simulink model "practice_main_pulse_inSimulink"  (R2019b)
settings: Solver=VariableStepAuto  StartTime=0.0  StopTime=0.1  RelTol=1e-3
InitFcn:
  | v_in=12;
undefined symbols (not defined in the file): plecs
settings Model: Creator=Nahid  LastModifiedBy=Nahid

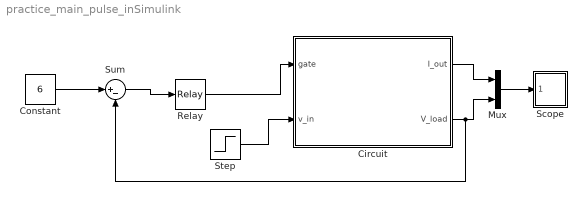
== system practice_main_pulse_inSimulink ==
  Circuit : Subsystem  LoadFcn=plecs('sl', 200);  InitFcn=plecs('sl', 214);  StartFcn=plecs('sl', 208);  StopFcn=plecs('sl', 209);  mask(PlecsCircuit){PLECSData=<binary blob, 2080 chars, not shown>}
      mask prompts: PLECSData "PLECS Data (Do not delete or modify!)"
      mask init:
      | % PLACE CUSTOM INITIALIZATIONS ABOVE
      | % DO NOT REMOVE
      | plecs('sl', 215);
      | % DO NOT REMOVE
      settings: CopyFcn=plecs('sl', 203);  DeleteFcn=plecs('sl', 205);  UndoDeleteFcn=plecs('sl', 206);  PreSaveFcn=plecs('sl', 211);  PostSaveFcn=plecs('sl', 201);  NameChangeFcn=plecs('sl', 210);  DestroyFcn=plecs('sl', 207);  PreCopyFcn=plecs('sl', 216);  OpenFcn=plecs('sl', 202);  ErrorFcn=plerrorfcn
      mask Help: web(['file:///' fullfile(plecsdoc, 'creatingacircuit.html')])
      mask Display: disp('PLECS\nCircuit')
  Constant : Constant  Value=6
  Mux : Mux  Inputs=2
  Relay : Relay  OnSwitchValue=0.2  OffSwitchValue=-0.2
  Scope : Subsystem  LoadFcn=plecs('sl', 300);  InitFcn=plecs('sl', 314);  StartFcn=plecs('sl', 308);  StopFcn=plecs('sl', 309);  mask{Settings=<binary blob, 1164 chars, not shown>}
      mask init:
      | plecs('sl', 315);
      settings: CopyFcn=plecs('sl', 303);  DeleteFcn=plecs('sl', 305);  UndoDeleteFcn=plecs('sl', 306);  PreSaveFcn=plecs('sl', 311);  NameChangeFcn=plecs('sl', 310);  DestroyFcn=plecs('sl', 307);  OpenFcn=plecs('sl', 302);  ErrorFcn=plerrorfcn
      mask Display: plot([0.1 0.9 0.9 0.1 0.1], [0.9 0.9 0.5 0.5 0.9])
  Step : Step  Time=0.05  Before=12  After=8  SampleTime=0
  Sum : Sum  Inputs=|+-
  wires:
  Circuit/1(I_out) -> Mux/1
  Circuit/2(V_load) -> Sum/2, Mux/2
  Mux/1 -> Scope/1(1)
  Constant/1 -> Sum/1
  Sum/1 -> Relay/1
  Relay/1 -> Circuit/1(gate)
  Step/1 -> Circuit/2(v_in)

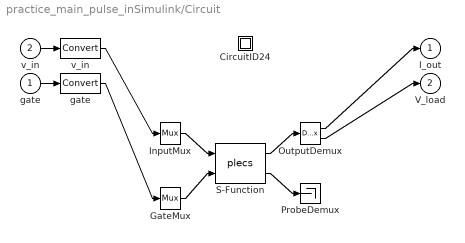
== system practice_main_pulse_inSimulink/Circuit ==
  gate : Inport  PortDimensions=1
  v_in : Inport  Port=2  PortDimensions=1
  " CircuitID24 " : Subsystem
  " GateMux " : Mux  Inputs=[ 1 ]
  " InputMux " : Mux  Inputs=[ 1 ]
  " OutputDemux " : Demux  Outputs=[ 1 1 ]
  " ProbeDemux " : Terminator
  " S-Function " : S-Function  FunctionName=plecs  SFunctionDeploymentMode=off  EnableBusSupport=off
  " gate " : DataTypeConversion  SaturateOnIntegerOverflow=on  RndMeth=Zero
  " v_in " : DataTypeConversion  SaturateOnIntegerOverflow=on  RndMeth=Zero
  I_out : Outport  PortDimensions=1
  V_load : Outport  Port=2  PortDimensions=1
  wires:
  " InputMux "/1 -> " S-Function "/1
  " GateMux "/1 -> " S-Function "/2
  " S-Function "/1 -> " OutputDemux "/1
  " S-Function "/2 -> " ProbeDemux "/1
  v_in/1 -> " v_in "/1
  " v_in "/1 -> " InputMux "/1
  gate/1 -> " gate "/1
  " gate "/1 -> " GateMux "/1
  " OutputDemux "/1 -> I_out/1
  " OutputDemux "/2 -> V_load/1

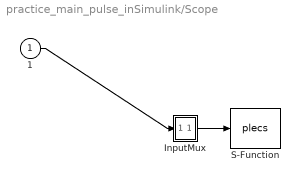
== system practice_main_pulse_inSimulink/Scope ==
  1 : Inport
  " InputMux " : Subsystem
      mask Display: disp('Mux')
  " S-Function " : S-Function  FunctionName=plecs  SFunctionDeploymentMode=off  EnableBusSupport=off
  wires:
  1/1 -> " InputMux "/1(In1)
  " InputMux "/1(Out) -> " S-Function "/1

== system practice_main_pulse_inSimulink/Circuit/ CircuitID24  ==

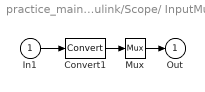
== system practice_main_pulse_inSimulink/Scope/ InputMux  ==
  In1 : Inport
  Convert1 : DataTypeConversion  SaturateOnIntegerOverflow=on  RndMeth=Zero
  Mux : Mux  Inputs=1
  Out : Outport
  wires:
  Convert1/1 -> Mux/1
  In1/1 -> Convert1/1
  Mux/1 -> Out/1
